simulink model "WMMSupportingForcesGP2020a"  (R2020a)
settings: Solver=ode23t  StartTime=0.0  StopTime=inf  FixedStep=.001  RelTol=1e-3  AbsTol=1e-3
InitFcn:
  | InitializeSimulationGP
  | SimulationParametersGP
values from neighbouring files (symbols this model uses):
  B11_r_B11C = [0.23805608; 0.13201777; 0]    [InitializeSimulationGP.m]
  B11_r_B11Tc1 = [L11; 0; 0]    [InitializeSimulationGP.m]
  B11_Rot_Tc1 = eye(3)    [InitializeSimulationGP.m]
  B11cI = [0.28426000 -0.06487287 0;         -0.06487287  0.54237481 0;                   0  0          0.67891020]    [InitializeSimulationGP.m]
  B12_r_B12C = [0.60504569; 0.27199376; 0.00002484]    [InitializeSimulationGP.m]
  B12_r_B12Tc2 = [L12;0;0]    [InitializeSimulationGP.m]
  B12_Rot_Tc2 = eye(3)    [InitializeSimulationGP.m]
  B12cI = [1.18803886 -2.36786418 0.00280315;          -2.36786418 6.31493281 0.00022322;           0.00280315 0.00022322 7.40915161]    [InitializeSimulationGP.m]
  B31_r_B31C = [0.35781210 0 0]    [InitializeSimulationGP.m]
  B31_Rot_B41 = eye(3)    [InitializeSimulationGP.m]
  B31cI = diag([0.03150902 0.90735702 0.90763033])    [InitializeSimulationGP.m]
  B32_r_B32C = [0.35781210 0 0]    [InitializeSimulationGP.m]
  B32_Rot_B42 = eye(3)    [InitializeSimulationGP.m]
  B32cI = diag([0.03150902 0.90735702 0.90763033])    [InitializeSimulationGP.m]
  B41_r_B41C = [0.55785997 0 0]    [InitializeSimulationGP.m]
  B41_r_B41Tc1 = [lc1;0;0]    [InitializeSimulationGP.m]
  B41cI = diag([0.00370720 0.55759812 0.55785997])    [InitializeSimulationGP.m]
  B42_r_B42C = [0.55785997 0 0]    [InitializeSimulationGP.m]
  B42_r_B42Tc2 = [lc2; 0; 0]    [InitializeSimulationGP.m]
  B42cI = diag([0.00370720 0.55759812 0.55785997])    [InitializeSimulationGP.m]
  B52_r_B52C = [0 0 0.56802906]    [InitializeSimulationGP.m]
  B52_r_B52P32 = [lc3; 0; 0]    [InitializeSimulationGP.m]
  B52_Rot_P32 = eye(3)    [InitializeSimulationGP.m]
  B52cI = diag([0.91789884, 0.91790043, 0.00091463])    [InitializeSimulationGP.m]
  Bc1_r_Bc1B11 = [L1; 0; 0]    [InitializeSimulationGP.m]
  Bc1_r_Bc1B31 = [0;0;0]    [InitializeSimulationGP.m]
  Bc1_r_Bc1C = [0.14178771; 0.16555780; 0]    [InitializeSimulationGP.m]
  Bc1_V = [0;0;0;0;0;0]    [InitializeSimulationGP.m]
  Bc1cI = [+5.892211080 +5.476111360 -0.000019630;          +5.476111360 +28.66965601 -0.000024550;          -0.000019630 -0.000024550 +29.78955950]    [InitializeSimulationGP.m]
  Bc2_r_Bc2B12 = [L2;0;0]    [InitializeSimulationGP.m]
  Bc2_r_Bc2B32 = [0;0;0]    [InitializeSimulationGP.m]
  Bc2_r_Bc2C = [0.54319901; 0.10543875; 0]    [InitializeSimulationGP.m]
  Bc2cI = [0.48071390 0.52924041 0;          0.52924041 5.80912352 0;              0      0          5.97255351]    [InitializeSimulationGP.m]
  BC_r_BCBM = [xCA; yCA; zCA]    [SimulationParametersGP.m]
  BC_Rot_BM = eye(3)    [SimulationParametersGP.m]
  BCI = diag([100 1200 1000])    [SimulationParametersGP.m]
  beta1 = atan2d(374.261,935)*pi/180    [InitializeSimulationGP.m]
  beta2 = atan2d(45.757,373.313)*pi/180    [InitializeSimulationGP.m]
  beta3 = atan2d(139.50,1132.19)*pi/180    [InitializeSimulationGP.m]
  beta4 = atan2d(88.061,296.198)*pi/180    [InitializeSimulationGP.m]
  betaGround = 1e6    (= 1000000)    [SimulationParametersGP.m]
  BFL = 0.05    [SimulationParametersGP.m]
  BFR = 0.05    [SimulationParametersGP.m]
  BM_r_BMBMp = [0;0;0]    [SimulationParametersGP.m]
  BM_Rot_BMp = [cos(gamma) -sin(gamma) 0; sin(gamma) cos(gamma) 0; 0 0 1]    [SimulationParametersGP.m]
  BMp_r_BMpBc1 = [0.185;0;0.205]    [InitializeSimulationGP.m]
  BMp_Rot_Bc1 = [cos(alpha1) -sin(alpha1)  0;                  0            0       -1;                sin(alpha1)  cos(alpha1)  0]    [InitializeSimulationGP.m]
  BRL = 0.05    [SimulationParametersGP.m]
  BRR = 0.05    [SimulationParametersGP.m]
  cc = 0.0    (= 0)    [SimulationParametersGP.m]
  D22F = [0;0;0;0;0;0]    [InitializeSimulationGP.m]
  dT = 0.01    [SimulationParametersGP.m]
  g0 = 9.8066    [SimulationParametersGP.m]
  ground_stiffness = 1e8    (= 100000000)    [SimulationParametersGP.m]
  l1 = 1.15-cc    (= 1.15)    [SimulationParametersGP.m]
  L1 = 1.0071227324212    (= 1.00712273242)    [InitializeSimulationGP.m]
  L11 = 0.37610632101293    (= 0.376106321013)    [InitializeSimulationGP.m]
  L12 = 0.30901132665325    (= 0.309011326653)    [InitializeSimulationGP.m]
  l2 = 1.15+cc    (= 1.15)    [SimulationParametersGP.m]
  L2 = 1.132185817991    (= 1.13218581799)    [InitializeSimulationGP.m]
  lc1 = 0.745    [InitializeSimulationGP.m]
  lc2 = 0.745    [InitializeSimulationGP.m]
  mB11 = 25.52660174    [InitializeSimulationGP.m]
  mB12 = 33.92850233    [InitializeSimulationGP.m]
  mB31 = 17.36281648    [InitializeSimulationGP.m]
  mB32 = 17.36281648    [InitializeSimulationGP.m]
  mB41 = 10.34519231    [InitializeSimulationGP.m]
  mB42 = 10.34519231    [InitializeSimulationGP.m]
  mB52 = 6.73059863    [InitializeSimulationGP.m]
  mBC = 2200    [SimulationParametersGP.m]
  mBc1 = 307.29601379    [InitializeSimulationGP.m]
  mBc2 = 54.58702836    [InitializeSimulationGP.m]
  mFL = 60    [SimulationParametersGP.m]
  mFR = 60    [SimulationParametersGP.m]
  mP22 = 9.26136143    [InitializeSimulationGP.m]
  mP32 = 570.18877059    [InitializeSimulationGP.m]
  mRR = 60    [SimulationParametersGP.m]
  mw = mFL    (= 60)    [SimulationParametersGP.m]
  P22_r_P22C = [0.62192523 0 0]    [InitializeSimulationGP.m]
  P22_Rot_B52 = eye(3)    [InitializeSimulationGP.m]
  P22cI = diag([0.00662754, 1.48387017, 1.48398069])    [InitializeSimulationGP.m]
  P32_r_P32C = [0.25466704; -0.13034397; -0.01302248]    [InitializeSimulationGP.m]
  P32_r_P32D22 = [0.40499744871392; -0.13130517281345; -0.013385243295654]    [InitializeSimulationGP.m]
  P32_Rot_D22 = [1 0 0;              0 0.9707729441837 0.23999977258512;              0 -0.23999977258512 0.9707729441837]    [InitializeSimulationGP.m]
  P32cI = [46.81220713 0.38607676 -0.00453819;          0.38607676 71.92201786 -1.14320993;          -0.00453819 -1.14320993 67.38128576]    [InitializeSimulationGP.m]
  R0FL = 0.35    [SimulationParametersGP.m]
  R0FR = 0.35    [SimulationParametersGP.m]
  R0RL = 0.35    [SimulationParametersGP.m]
  R0RR = 0.35    [SimulationParametersGP.m]
  Rw = R0FL    (= 0.35)    [SimulationParametersGP.m]
  Tc1_r_Tc1Bc2 = [0.098495302558553; 0.01838181329939; 0]    [InitializeSimulationGP.m]
  Tc1_Rot_Bc2 = [cos(alpha2) -sin(alpha2) 0;                sin(alpha2)  cos(alpha2) 0;                0            0           1]    [InitializeSimulationGP.m]
  Tc2_r_Tc2P22 = [-0.048858374920227;0.36587359346146;0.035276938723102]    [InitializeSimulationGP.m]
  Tc2_Rot_P22 = [0.95853460763586 -0.27664713597974  0.0683942111482;                0.28497614981675  0.93051946315663 -0.23004808784757;                0                 0.23999977258511  0.9707729441837]    [InitializeSimulationGP.m]
  Th1A = 10*pi/180    (= 0.174532925199)    [InitializeSimulationGP.m]
  Th1B = 20*pi/180    (= 0.349065850399)    [InitializeSimulationGP.m]
  Th1f = 1    [InitializeSimulationGP.m]
  Th2A = 15*pi/180    (= 0.261799387799)    [InitializeSimulationGP.m]
  Th2B = -70*pi/180    (= -1.2217304764)    [InitializeSimulationGP.m]
  Th2f = 2    [InitializeSimulationGP.m]
  w = wFL    (= 0.875)    [SimulationParametersGP.m]
  W_r_WBc1 = [0.185;0;0.205]    [InitializeSimulationGP.m]
  W_Rot_Bc1 = [cos(alpha1) -sin(alpha1)  0;                  0            0       -1;                sin(alpha1)  cos(alpha1)  0]    [InitializeSimulationGP.m]
  x10 = 0.83    [InitializeSimulationGP.m]
  x20 = 0.83    [InitializeSimulationGP.m]
  x3A = 0.2    [InitializeSimulationGP.m]
  x3B = 0.3    [InitializeSimulationGP.m]
  x3f = 1    [InitializeSimulationGP.m]
  xCA = 0.5    [SimulationParametersGP.m]
  xf = [1;0;0;0;0;0]    [InitializeSimulationGP.m]
  yCA = 0    [SimulationParametersGP.m]
  zC = 0.45    [SimulationParametersGP.m]
  zCA = .25    (= 0.25)    [SimulationParametersGP.m]
  ztau = [0;0;0;0;0;1]    [InitializeSimulationGP.m]
undefined symbols (not defined in the file or in its folder): alphaFL_meas, alphaFR_meas, alphaRL_meas, alphaRR_meas, B11_V, B11Ftot, B12_U_Tc2, B12_V, B12Ftot, B31_r_B31B41, B31_V, B31FTot, B32_r_B32B42, B32_U_B42, B32_V, B32FTot, B41_V, B41FTot, B42_Rot_Tc2, B42_U_Tc2, B42_V, B42FTot, B52_U_P32, B52_V, B52Ftot, Bc1Tot, Bc2_Rot_B12, Bc2_Rot_B32, Bc2_U_B12, Bc2_U_B32, Bc2_V, Bc2Tot, betaC_meas, D22_V, deltaFL_cmd, deltaFL_meas, deltaFR_cmd, deltaFR_meas, deltaRL_cmd, deltaRL_meas, deltaRR_cmd, deltaRR_meas, dOmegaFL_meas, dOmegaFR_meas, dOmegaRL_meas, dOmegaRR_meas, dPsi_meas, dq1, dq11, dq12, dq2, dq21, dq22, dx1, dx2, Floor, FTot_S1, FTot_S2P, FTot_S2R, FzFL ... (+63)
libraries: sm_lib x94, nesl_utility x63, simulink x5
(part 8 of 11)

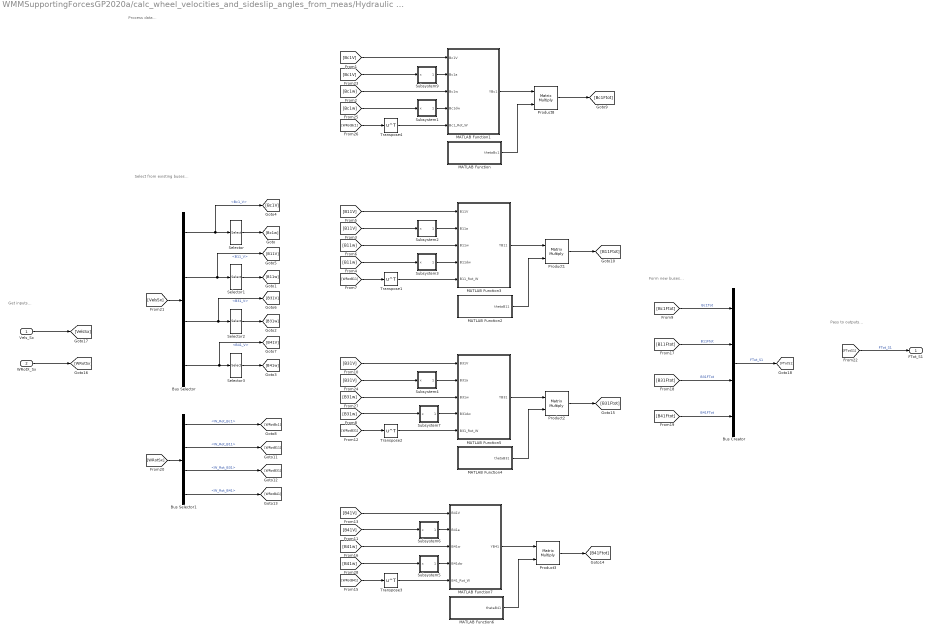
== system WMMSupportingForcesGP2020a/calc_wheel_velocities_and_sideslip_angles_from_meas/Hydraulic manipulator, calculation/AnalyticTotalForces/Structure 1 ==
  note: Pass to outputs...
  note: Get inputs...
  note: Process data...
  note: Form new buses...
  note: Select from existing buses...
  Vels_Sx : Inport
  WRotX_Sx : Inport  Port=2
  Bus Creator : BusCreator  Inputs=Bc1Tot,B11Ftot,B31FTot,B41FTot
  Bus Selector : BusSelector  OutputSignals=Vels_S1.Bc1_V,Vels_S1.B11_V,Vels_S1.B31_V,Vels_S1.B41_V
  Bus Selector1 : BusSelector  OutputSignals=WRotX_S1.W_Rot_Bc1,WRotX_S1.W_Rot_B11,WRotX_S1.W_Rot_B31,WRotX_S1.W_Rot_B41
  MATLAB Function : MATLAB Function  TreatAsAtomicUnit=on
  MATLAB Function1 : MATLAB Function  TreatAsAtomicUnit=on
  MATLAB Function2 : MATLAB Function  TreatAsAtomicUnit=on
  MATLAB Function3 : MATLAB Function  TreatAsAtomicUnit=on
  MATLAB Function4 : MATLAB Function  TreatAsAtomicUnit=on
  MATLAB Function5 : MATLAB Function  TreatAsAtomicUnit=on
  MATLAB Function6 : MATLAB Function  TreatAsAtomicUnit=on
  MATLAB Function7 : MATLAB Function  TreatAsAtomicUnit=on
  Product{1..3,8} (4 alike) : Product  Multiplication=Matrix(*)
  Selector{,1..3} (4 alike) : Selector  InputPortWidth=6  IndexOptions=Index vector (dialog)  Indices=[4 5 6]  OutputSizes=1
  Subsystem1 : Subsystem
  Subsystem2 : Subsystem
  Subsystem3 : Subsystem
  Subsystem4 : Subsystem
  Subsystem5 : Subsystem
  Subsystem6 : Subsystem
  Subsystem7 : Subsystem
  Subsystem9 : Subsystem
  Transpose{1..4} (4 alike) : Math  Operator=transpose  SaturateOnIntegerOverflow=on
  FTot_S1 : Outport
  wires:
  Bus Selector/4 -> Selector3/1, [B41V]  "<B41_V>"
  Bus Selector1/3 -> [WRotB31]  "<W_Rot_B31>"
  Bus Selector1/1 -> [WRotBc1]  "<W_Rot_Bc1>"
  [B11Ftot] -> Bus Creator/2  "B11Ftot"
  [WRotB31] -> Transpose2/1
  Selector/1 -> [Bc1w]
  Selector3/1 -> [B41w]
  Bus Selector/3 -> Selector2/1, [B31V]  "<B31_V>"
  [B31Ftot] -> Bus Creator/3  "B31FTot"
  Bus Selector/1 -> Selector/1, [Bc1V]  "<Bc1_V>"
  Bus Selector/2 -> Selector1/1, [B11V]  "<B11_V>"
  [B41Ftot] -> Bus Creator/4  "B41FTot"
  Selector2/1 -> [B31w]
  [Bc1Ftot] -> Bus Creator/1  "Bc1Tot"
  Bus Selector1/2 -> [WRotB11]  "<W_Rot_B11>"
  [WRotB11] -> Transpose1/1
  Bus Selector1/4 -> [WRotB41]  "<W_Rot_B41>"
  WRotX_Sx/1 -> [WRotSx]
  [WRotSx] -> Bus Selector1/1
  Vels_Sx/1 -> [VelsSx]
  [VelsSx] -> Bus Selector/1
  Bus Creator/1 -> [FTotS1]  "FTot_S1"
  [FTotS1] -> FTot_S1/1  "FTot_S1"
  Selector1/1 -> [B11w]
  [WRotBc1] -> Transpose4/1
  Transpose4/1 -> MATLAB Function1/5(Bc1_Rot_W)
  Subsystem1/1(dx/dt) -> MATLAB Function1/4(Bc1dw)
  [Bc1w] -> Subsystem1/1(x)
  [Bc1V] -> Subsystem9/1(x)
  Subsystem9/1(dx/dt) -> MATLAB Function1/2(Bc1a)
  MATLAB Function1/1(YBc1) -> Product8/1
  MATLAB Function/1(thetaBc1) -> Product8/2
  Product8/1 -> [Bc1Ftot]
  [Bc1V] -> MATLAB Function1/1(Bc1V)
  [Bc1w] -> MATLAB Function1/3(Bc1w)
  [B11w] -> MATLAB Function3/3(B11w)
  [B11V] -> MATLAB Function3/1(B11V)
  MATLAB Function2/1(thetaB11) -> Product1/2
  MATLAB Function3/1(YB11) -> Product1/1
  Subsystem2/1(dx/dt) -> MATLAB Function3/2(B11a)
  [B11V] -> Subsystem2/1(x)
  [B11w] -> Subsystem3/1(x)
  Subsystem3/1(dx/dt) -> MATLAB Function3/4(B11dw)
  Transpose1/1 -> MATLAB Function3/5(B11_Rot_W)
  Product1/1 -> [B11Ftot]
  Product2/1 -> [B31Ftot]
  Transpose2/1 -> MATLAB Function5/5(B31_Rot_W)
  Subsystem7/1(dx/dt) -> MATLAB Function5/4(B31dw)
  [B31w] -> Subsystem7/1(x)
  [B31V] -> Subsystem4/1(x)
  Subsystem4/1(dx/dt) -> MATLAB Function5/2(B31a)
  MATLAB Function5/1(YB31) -> Product2/1
  MATLAB Function4/1(thetaB31) -> Product2/2
  [B31V] -> MATLAB Function5/1(B31V)
  [B31w] -> MATLAB Function5/3(B31w)
  [B41w] -> MATLAB Function7/3(B41w)
  [B41V] -> MATLAB Function7/1(B41V)
  MATLAB Function6/1(thetaB41) -> Product3/2
  MATLAB Function7/1(YB41) -> Product3/1
  Subsystem6/1(dx/dt) -> MATLAB Function7/2(B41a)
  [B41V] -> Subsystem6/1(x)
  [B41w] -> Subsystem5/1(x)
  Subsystem5/1(dx/dt) -> MATLAB Function7/4(B41dw)
  Transpose3/1 -> MATLAB Function7/5(B41_Rot_W)
  Product3/1 -> [B41Ftot]
  [WRotB41] -> Transpose3/1

== system WMMSupportingForcesGP2020a/calc_wheel_velocities_and_sideslip_angles_from_meas/Hydraulic manipulator, calculation/AnalyticTotalForces/Structure 2 (Prismatic segment) ==
  note: Select from existing buses...
  note: Form new buses...
  note: Get inputs...
  note: Pass to outputs...
  note: Process data...
  Vels_Sx : Inport
  WRotX_Sx : Inport  Port=2
  Bus Creator : BusCreator  Inputs=P22FTot,B52Ftot,P32FTot
  Bus Selector : BusSelector  OutputSignals=Vels_S2R.P22_V,Vels_S2P.B52_V,Vels_S2P.P32_V
  Bus Selector1 : BusSelector  OutputSignals=WRotX_S2R.W_Rot_P22,WRotX_S2P.W_Rot_B52,WRotX_S2P.W_Rot_P32
  MATLAB Function1 : MATLAB Function  TreatAsAtomicUnit=on
  MATLAB Function2 : MATLAB Function  TreatAsAtomicUnit=on
  MATLAB Function3 : MATLAB Function  TreatAsAtomicUnit=on
  MATLAB Function4 : MATLAB Function  TreatAsAtomicUnit=on
  MATLAB Function6 : MATLAB Function  TreatAsAtomicUnit=on
  MATLAB Function7 : MATLAB Function  TreatAsAtomicUnit=on
  Product1 : Product  Multiplication=Matrix(*)
  Product2 : Product  Multiplication=Matrix(*)
  Product3 : Product  Multiplication=Matrix(*)
  Selector : Selector  InputPortWidth=6  IndexOptions=Index vector (dialog)  Indices=[4 5 6]  OutputSizes=1
  Selector1 : Selector  InputPortWidth=6  IndexOptions=Index vector (dialog)  Indices=[4 5 6]  OutputSizes=1
  Selector2 : Selector  InputPortWidth=6  IndexOptions=Index vector (dialog)  Indices=[4 5 6]  OutputSizes=1
  Subsystem1 : Subsystem
  Subsystem2 : Subsystem
  Subsystem3 : Subsystem
  Subsystem4 : Subsystem
  Subsystem5 : Subsystem
  Subsystem6 : Subsystem
  Transpose : Math  Operator=transpose  SaturateOnIntegerOverflow=on
  Transpose1 : Math  Operator=transpose  SaturateOnIntegerOverflow=on
  Transpose2 : Math  Operator=transpose  SaturateOnIntegerOverflow=on
  FTot_S2P : Outport
  wires:
  [FTotS2P] -> FTot_S2P/1  "FTot_S2P"
  WRotX_Sx/1 -> [WRotSx]
  Vels_Sx/1 -> [VelsSx]
  Product3/1 -> [P32Ftot]
  Bus Selector1/3 -> [WRotP32]  "<W_Rot_P32>"
  [VelsSx] -> Bus Selector/1
  Product2/1 -> [B52Ftot]
  Bus Selector1/1 -> [WRotP22]  "<W_Rot_P22>"
  [B52Ftot] -> Bus Creator/2  "B52Ftot"
  Product1/1 -> [P22Ftot]
  [WRotP22] -> Transpose/1
  [WRotP32] -> Transpose2/1
  Selector/1 -> [P22w]
  Bus Creator/1 -> [FTotS2P]
  [WRotSx] -> Bus Selector1/1
  Selector1/1 -> [B52w]
  [P32Ftot] -> Bus Creator/3  "P32FTot"
  Selector2/1 -> [P32w]
  [P22Ftot] -> Bus Creator/1  "P22FTot"
  Bus Selector1/2 -> [WRotB52]  "<W_Rot_B52>"
  Bus Selector/1 -> [P22V], Selector/1  "<P22_V>"
  Bus Selector/3 -> [P32V], Selector2/1  "<P32_V>"
  Bus Selector/2 -> [B52V], Selector1/1  "<B52_V>"
  [P22V] -> MATLAB Function7/1(P22V)
  Transpose/1 -> MATLAB Function7/5(P22_Rot_W)
  [P22V] -> Subsystem2/1(x)
  [P22w] -> Subsystem1/1(x)
  MATLAB Function7/1(YP22) -> Product1/1
  Subsystem1/1(dx/dt) -> MATLAB Function7/4(P22dw)
  MATLAB Function6/1(thetaP22) -> Product1/2
  Subsystem2/1(dx/dt) -> MATLAB Function7/2(P22a)
  [P22w] -> MATLAB Function7/3(P22w)
  MATLAB Function1/1(thetaB52) -> Product2/2
  MATLAB Function2/1(YB52) -> Product2/1
  [WRotB52] -> Transpose1/1
  [B52V] -> MATLAB Function2/1(B52V)
  [B52V] -> Subsystem3/1(x)
  Subsystem3/1(dx/dt) -> MATLAB Function2/2(B52a)
  [B52w] -> MATLAB Function2/3(B52w)
  [B52w] -> Subsystem4/1(x)
  Subsystem4/1(dx/dt) -> MATLAB Function2/4(B52dw)
  Transpose1/1 -> MATLAB Function2/5(B52_Rot_W)
  Transpose2/1 -> MATLAB Function4/5(P32_Rot_W)
  Subsystem6/1(dx/dt) -> MATLAB Function4/4(P32dw)
  [P32w] -> Subsystem6/1(x)
  [P32w] -> MATLAB Function4/3(P32w)
  Subsystem5/1(dx/dt) -> MATLAB Function4/2(P32a)
  [P32V] -> Subsystem5/1(x)
  [P32V] -> MATLAB Function4/1(P32V)
  MATLAB Function4/1(YP32) -> Product3/1
  MATLAB Function3/1(thetaP32) -> Product3/2

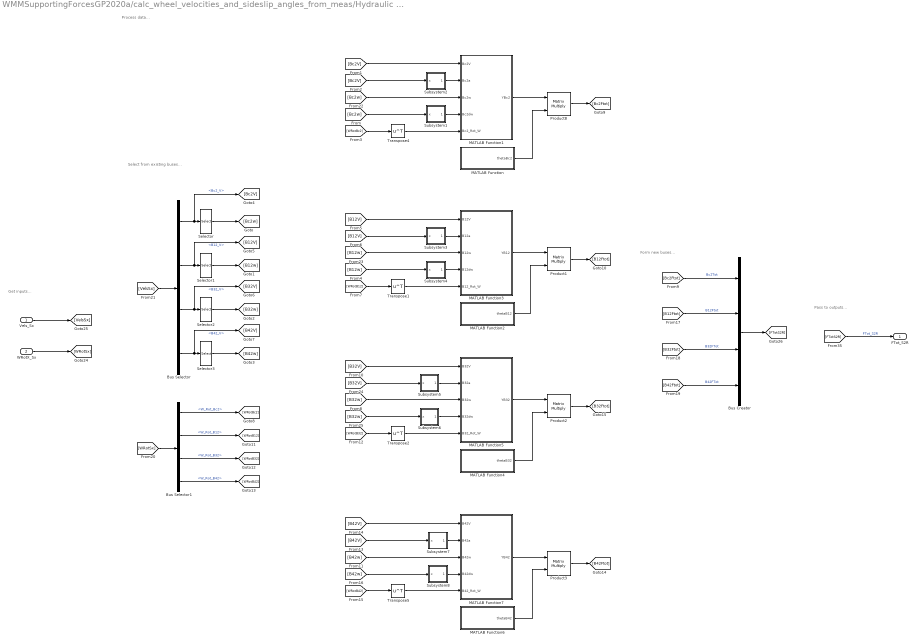
== system WMMSupportingForcesGP2020a/calc_wheel_velocities_and_sideslip_angles_from_meas/Hydraulic manipulator, calculation/AnalyticTotalForces/Structure 2 (Revolute segment) ==
  note: Process data...
  note: Pass to outputs...
  note: Get inputs...
  note: Form new buses...
  note: Select from existing buses...
  Vels_Sx : Inport
  WRotX_Sx : Inport  Port=2
  Bus Creator : BusCreator  Inputs=Bc2Tot,B12Ftot,B32FTot,B42FTot
  Bus Selector : BusSelector  OutputSignals=Vels_S1.Bc2_V,Vels_S2R.B12_V,Vels_S2R.B32_V,Vels_S2R.B42_V
  Bus Selector1 : BusSelector  OutputSignals=WRotX_S1.W_Rot_Bc2,WRotX_S2R.W_Rot_B12,WRotX_S2R.W_Rot_B32,WRotX_S2R.W_Rot_B42
  MATLAB Function : MATLAB Function  TreatAsAtomicUnit=on
  MATLAB Function1 : MATLAB Function  TreatAsAtomicUnit=on
  MATLAB Function2 : MATLAB Function  TreatAsAtomicUnit=on
  MATLAB Function3 : MATLAB Function  TreatAsAtomicUnit=on
  MATLAB Function4 : MATLAB Function  TreatAsAtomicUnit=on
  MATLAB Function5 : MATLAB Function  TreatAsAtomicUnit=on
  MATLAB Function6 : MATLAB Function  TreatAsAtomicUnit=on
  MATLAB Function7 : MATLAB Function  TreatAsAtomicUnit=on
  Product{1..3,8} (4 alike) : Product  Multiplication=Matrix(*)
  Selector{,1..3} (4 alike) : Selector  InputPortWidth=6  IndexOptions=Index vector (dialog)  Indices=[4 5 6]  OutputSizes=1
  Subsystem1 : Subsystem
  Subsystem2 : Subsystem
  Subsystem3 : Subsystem
  Subsystem4 : Subsystem
  Subsystem5 : Subsystem
  Subsystem6 : Subsystem
  Subsystem7 : Subsystem
  Subsystem8 : Subsystem
  Transpose{1..2,4..5} (4 alike) : Math  Operator=transpose  SaturateOnIntegerOverflow=on
  FTot_S2R : Outport
  wires:
  Bus Selector1/4 -> [WRotB42]  "<W_Rot_B42>"
  [WRotB12] -> Transpose1/1
  Bus Selector1/2 -> [WRotB12]  "<W_Rot_B12>"
  [WRotB42] -> Transpose5/1
  [Bc2Ftot] -> Bus Creator/1  "Bc2Tot"
  Selector2/1 -> [B32w]
  [B42Ftot] -> Bus Creator/4  "B42FTot"
  Bus Selector/2 -> Selector1/1, [B12V]  "<B12_V>"
  Bus Selector/1 -> Selector/1, [Bc2V]  "<Bc2_V>"
  [B32Ftot] -> Bus Creator/3  "B32FTot"
  Bus Selector/3 -> Selector2/1, [B32V]  "<B32_V>"
  Selector1/1 -> [B12w]
  [WRotSx] -> Bus Selector1/1
  Selector3/1 -> [B42w]
  Bus Creator/1 -> [FTotS2R]
  Selector/1 -> [Bc2w]
  [WRotB32] -> Transpose2/1
  Product3/1 -> [B42Ftot]
  Product8/1 -> [Bc2Ftot]
  [B12Ftot] -> Bus Creator/2  "B12Ftot"
  Bus Selector1/1 -> [WRotBc2]  "<W_Rot_Bc2>"
  [VelsSx] -> Bus Selector/1
  Bus Selector1/3 -> [WRotB32]  "<W_Rot_B32>"
  Bus Selector/4 -> Selector3/1, [B42V]  "<B42_V>"
  Vels_Sx/1 -> [VelsSx]
  WRotX_Sx/1 -> [WRotSx]
  [FTotS2R] -> FTot_S2R/1  "FTot_S2R"
  [Bc2w] -> Subsystem1/1(x)
  [Bc2w] -> MATLAB Function1/3(Bc2w)
  [WRotBc2] -> Transpose4/1
  Transpose4/1 -> MATLAB Function1/5(Bc2_Rot_W)
  Subsystem1/1(dx/dt) -> MATLAB Function1/4(Bc2dw)
  [Bc2V] -> MATLAB Function1/1(Bc2V)
  MATLAB Function/1(thetaBc2) -> Product8/2
  [Bc2V] -> Subsystem2/1(x)
  MATLAB Function1/1(YBc2) -> Product8/1
  Subsystem2/1(dx/dt) -> MATLAB Function1/2(Bc2a)
  Subsystem3/1(dx/dt) -> MATLAB Function3/2(B12a)
  MATLAB Function3/1(YB12) -> Product1/1
  [B12V] -> Subsystem3/1(x)
  MATLAB Function2/1(thetaB12) -> Product1/2
  [B12V] -> MATLAB Function3/1(B12V)
  Subsystem4/1(dx/dt) -> MATLAB Function3/4(B12dw)
  Transpose1/1 -> MATLAB Function3/5(B12_Rot_W)
  [B12w] -> MATLAB Function3/3(B12w)
  [B12w] -> Subsystem4/1(x)
  Product1/1 -> [B12Ftot]
  [B32w] -> Subsystem6/1(x)
  [B32w] -> MATLAB Function5/3(B32w)
  Subsystem6/1(dx/dt) -> MATLAB Function5/4(B32dw)
  [B32V] -> MATLAB Function5/1(B32V)
  MATLAB Function4/1(thetaB32) -> Product2/2
  [B32V] -> Subsystem5/1(x)
  MATLAB Function5/1(YB32) -> Product2/1
  Subsystem5/1(dx/dt) -> MATLAB Function5/2(B32a)
  Transpose2/1 -> MATLAB Function5/5(B32_Rot_W)
  Product2/1 -> [B32Ftot]
  Transpose5/1 -> MATLAB Function7/5(B42_Rot_W)
  Subsystem7/1(dx/dt) -> MATLAB Function7/2(B42a)
  MATLAB Function7/1(YB42) -> Product3/1
  [B42V] -> Subsystem7/1(x)
  MATLAB Function6/1(thetaB42) -> Product3/2
  [B42V] -> MATLAB Function7/1(B42V)
  Subsystem8/1(dx/dt) -> MATLAB Function7/4(B42dw)
  [B42w] -> MATLAB Function7/3(B42w)
  [B42w] -> Subsystem8/1(x)

== system WMMSupportingForcesGP2020a/calc_wheel_velocities_and_sideslip_angles_from_meas/Hydraulic manipulator, calculation/AnalyticVelocities/Structure 1 ==
  note: Pass to outputs...
  note: Process data...
  note: Calculate geometric properties of the closed kinematic chain 1...
  note: Get inputs...
  note: Form relevant position vectors...
  note: Form relevant rotation matrices...
  note: Form relevant velocity/force transformation matrices...
  note: Form relevant linear/angular velocities...
  q1[rad] : Inport  Unit=rad
  W_Rot_Bc1 : Inport  Port=2
  Bc1_V : Inport  Port=3  PortDimensions=[6 1]
  GeomPropS1 : Subsystem
  PosVecsS1 : Subsystem
  RotMatsS1 : Subsystem
  UMatsS1 : Subsystem
  VelsS1 : Subsystem
  Geom_S1 : Outport
  PosVecs_S1 : Outport  Port=2
  WRotX_S1 : Outport  Port=3
  Vels_S1 : Outport  Port=4
  UMat_S1 : Outport  Port=5
  wires:
  GeomPropS1/1(GeomProp_S1) -> [GeomS1]
  [GeomS1] -> PosVecsS1/1(GeomProp_CC1)
  [GeomS1] -> RotMatsS1/1(GeomProp_S1)
  [GeomS1] -> VelsS1/1(GeomProp_S1)
  RotMatsS1/1(RotMats_S1) -> [RotMatsS1]
  [RotMatsS1] -> UMatsS1/2(RotMats_S1)
  PosVecsS1/1(PosVecs_S1) -> [PosVecsS1]
  [PosVecsS1] -> UMatsS1/1(PosVecs_S1)
  [GeomS1] -> Geom_S1/1
  VelsS1/1(Vels_S1) -> [VelsS1]
  [VelsS1] -> Vels_S1/1
  UMatsS1/1(UMat_S1) -> [UMatsS1]
  [UMatsS1] -> VelsS1/2(UMats_S1)
  Bc1_V/1 -> [Bc1V]  "Bc1V"
  [Bc1V] -> VelsS1/3(Bc1_V)
  W_Rot_Bc1/1 -> [WRotBc1]  "WRotBc1"
  [WRotBc1] -> RotMatsS1/2(WRotBc1)
  [UMatsS1] -> UMat_S1/1
  RotMatsS1/2(WRotX_S1) -> [WRotXS1]
  [WRotXS1] -> WRotX_S1/1
  q1[rad]/1 -> [q1]  "q1"
  [q1] -> GeomPropS1/1(q1)
  [PosVecsS1] -> PosVecs_S1/1

== system WMMSupportingForcesGP2020a/calc_wheel_velocities_and_sideslip_angles_from_meas/Hydraulic manipulator, calculation/AnalyticVelocities/Structure 2 (Prismatic segment) ==
  note: Pass to outputs...
  note: Get inputs...
  note: Process data...
  x3 : Inport
  WRotX_S2R : Inport  Port=2
  Vels_S2R : Inport  Port=3
  GeomPropS2P : Subsystem
  PosVecsS2P : Subsystem
  RotMatsS2P : Subsystem
  UMatsS2P : Subsystem
  VelsS2P : Subsystem
  GeomProp_S2P : Outport
  PosVecs_S2P : Outport  Port=2
  WRotX_S2P : Outport  Port=3
  Vels_S2P : Outport  Port=4
  UMats_S2P : Outport  Port=5
  wires:
  x3/1 -> [x3]
  Vels_S2R/1 -> [VelsS2R]
  WRotX_S2R/1 -> [WRotXS2R]
  GeomPropS2P/1(GeomProp_S2P) -> [GeomS2P]
  [GeomS2P] -> GeomProp_S2P/1
  [x3] -> GeomPropS2P/1(x3)
  PosVecsS2P/1(PosVecsS2P) -> [PosVecsS2P]
  [x3] -> PosVecsS2P/1(x3)
  [PosVecsS2P] -> PosVecs_S2P/1
  RotMatsS2P/2(WRotX_S2P) -> [WRotXS2P]
  [WRotXS2R] -> RotMatsS2P/1(WRotX_S2R)
  [WRotXS2P] -> WRotX_S2P/1
  RotMatsS2P/1(RotMats_S2P) -> [RotMatsS2P]
  [PosVecsS2P] -> UMatsS2P/1(PosVecs_S2P)
  [RotMatsS2P] -> UMatsS2P/2(RotMats_S2P)
  UMatsS2P/1(UMats_S2P) -> [UMatsS2P]
  [UMatsS2P] -> UMats_S2P/1
  [VelsS2R] -> VelsS2P/3(Vels_S2R)
  [GeomS2P] -> VelsS2P/1(GeomProp_S2P)
  [UMatsS2P] -> VelsS2P/2(UMats_S2P)
  VelsS2P/1(Vels_S2P) -> [VelsS2P]
  [VelsS2P] -> Vels_S2P/1

== system WMMSupportingForcesGP2020a/calc_wheel_velocities_and_sideslip_angles_from_meas/Hydraulic manipulator, calculation/AnalyticVelocities/Structure 2 (Revolute segment) ==
  note: Pass to outputs...
  note: Process data...
  note: Get inputs...
  q2[rad] : Inport
  WRotX_S1 : Inport  Port=2
  Vels_S1 : Inport  Port=3
  GeomPropS2R : Subsystem
  PosVecsS2R : Subsystem
  RotMatsS2R : Subsystem
  UMatS2R : Subsystem
  VelsS2R : Subsystem
  GeomProp_S2R : Outport
  PosVecs_S2R : Outport  Port=2
  WRotX_S2R : Outport  Port=3
  Vels_S2R : Outport  Port=4
  UMats_S2R : Outport  Port=5
  wires:
  [GeomS2R] -> VelsS2R/1(GeomProp_CC2)
  [GeomS2R] -> RotMatsS2R/1(GeomProp_CC2)
  [GeomS2R] -> PosVecsS2R/1(GeomProp_S2R)
  GeomPropS2R/1(GeomProp_S2R) -> [GeomS2R]
  [q2] -> GeomPropS2R/1(q2)
  [GeomS2R] -> GeomProp_S2R/1  "GeomS2R"
  RotMatsS2R/1(RotMats_S2) -> [RotMatsS2R]
  q2[rad]/1 -> [q2]  "q2"
  PosVecsS2R/1(PosVecs_S2) -> [PosVecsS2R]
  [PosVecsS2R] -> UMatS2R/1(PosVecs_S2)
  [PosVecsS2R] -> PosVecs_S2R/1  "PosVecsS2R"
  [RotMatsS2R] -> UMatS2R/2(RotMats_S2)
  UMatS2R/1(UMatS2) -> [UMatsS2R]
  [UMatsS2R] -> VelsS2R/2(UMats_S2)
  [UMatsS2R] -> UMats_S2R/1  "UMatsS2R"
  RotMatsS2R/2(WRotX_S2) -> [WRotXS2R]
  [WRotXS2R] -> WRotX_S2R/1  "WRotXS2R"
  Vels_S1/1 -> [VelsS1]  "Vels_S1"
  [VelsS1] -> VelsS2R/3(Vels_S1)
  WRotX_S1/1 -> [WRotXS1]  "WRotX_S1"
  [WRotXS1] -> RotMatsS2R/2(WRotX_S1)
  VelsS2R/1(Vels_S2) -> [VelsS2R]
  [VelsS2R] -> Vels_S2R/1  "VelsS2R"

== system WMMSupportingForcesGP2020a/calc_wheel_velocities_and_sideslip_angles_from_meas/Hydraulic manipulator, calculation/AnalyticTotalForces/Structure 1/Subsystem1 ==
  x : Inport
  Demux : Demux  Outputs=3
  Mux : Mux  Inputs=3
  Subsystem1 : Subsystem
  Subsystem2 : Subsystem
  Subsystem3 : Subsystem
  dx/dt : Outport
  wires:
  x/1 -> Demux/1
  Demux/3 -> Subsystem3/1(x)
  Demux/2 -> Subsystem2/1(x)
  Demux/1 -> Subsystem1/1(x)
  Subsystem3/1(dx/dt) -> Mux/3
  Subsystem2/1(dx/dt) -> Mux/2
  Subsystem1/1(dx/dt) -> Mux/1
  Mux/1 -> dx/dt/1

== system WMMSupportingForcesGP2020a/calc_wheel_velocities_and_sideslip_angles_from_meas/Hydraulic manipulator, calculation/AnalyticTotalForces/Structure 1/Subsystem2 ==
  x : Inport
  Demux : Demux  Outputs=6
  Mux : Mux  Inputs=6
  Subsystem1 : Subsystem
  Subsystem2 : Subsystem
  Subsystem3 : Subsystem
  Subsystem4 : Subsystem
  Subsystem5 : Subsystem
  Subsystem6 : Subsystem
  dx/dt : Outport
  wires:
  x/1 -> Demux/1
  Demux/6 -> Subsystem6/1(x)
  Demux/5 -> Subsystem5/1(x)
  Demux/4 -> Subsystem4/1(x)
  Demux/3 -> Subsystem3/1(x)
  Demux/2 -> Subsystem2/1(x)
  Demux/1 -> Subsystem1/1(x)
  Subsystem6/1(dx/dt) -> Mux/6
  Subsystem5/1(dx/dt) -> Mux/5
  Subsystem4/1(dx/dt) -> Mux/4
  Subsystem3/1(dx/dt) -> Mux/3
  Subsystem2/1(dx/dt) -> Mux/2
  Subsystem1/1(dx/dt) -> Mux/1
  Mux/1 -> dx/dt/1

== system WMMSupportingForcesGP2020a/calc_wheel_velocities_and_sideslip_angles_from_meas/Hydraulic manipulator, calculation/AnalyticTotalForces/Structure 1/Subsystem3 ==
  x : Inport
  Demux : Demux  Outputs=3
  Mux : Mux  Inputs=3
  Subsystem1 : Subsystem
  Subsystem2 : Subsystem
  Subsystem3 : Subsystem
  dx/dt : Outport
  wires:
  x/1 -> Demux/1
  Demux/3 -> Subsystem3/1(x)
  Demux/2 -> Subsystem2/1(x)
  Demux/1 -> Subsystem1/1(x)
  Subsystem3/1(dx/dt) -> Mux/3
  Subsystem2/1(dx/dt) -> Mux/2
  Subsystem1/1(dx/dt) -> Mux/1
  Mux/1 -> dx/dt/1

== system WMMSupportingForcesGP2020a/calc_wheel_velocities_and_sideslip_angles_from_meas/Hydraulic manipulator, calculation/AnalyticTotalForces/Structure 1/Subsystem4 ==
  x : Inport
  Demux : Demux  Outputs=6
  Mux : Mux  Inputs=6
  Subsystem1 : Subsystem
  Subsystem2 : Subsystem
  Subsystem3 : Subsystem
  Subsystem4 : Subsystem
  Subsystem5 : Subsystem
  Subsystem6 : Subsystem
  dx/dt : Outport
  wires:
  x/1 -> Demux/1
  Demux/6 -> Subsystem6/1(x)
  Demux/5 -> Subsystem5/1(x)
  Demux/4 -> Subsystem4/1(x)
  Demux/3 -> Subsystem3/1(x)
  Demux/2 -> Subsystem2/1(x)
  Demux/1 -> Subsystem1/1(x)
  Subsystem6/1(dx/dt) -> Mux/6
  Subsystem5/1(dx/dt) -> Mux/5
  Subsystem4/1(dx/dt) -> Mux/4
  Subsystem3/1(dx/dt) -> Mux/3
  Subsystem2/1(dx/dt) -> Mux/2
  Subsystem1/1(dx/dt) -> Mux/1
  Mux/1 -> dx/dt/1

== system WMMSupportingForcesGP2020a/calc_wheel_velocities_and_sideslip_angles_from_meas/Hydraulic manipulator, calculation/AnalyticTotalForces/Structure 1/Subsystem5 ==
  x : Inport
  Demux : Demux  Outputs=3
  Mux : Mux  Inputs=3
  Subsystem1 : Subsystem
  Subsystem2 : Subsystem
  Subsystem3 : Subsystem
  dx/dt : Outport
  wires:
  x/1 -> Demux/1
  Demux/3 -> Subsystem3/1(x)
  Demux/2 -> Subsystem2/1(x)
  Demux/1 -> Subsystem1/1(x)
  Subsystem3/1(dx/dt) -> Mux/3
  Subsystem2/1(dx/dt) -> Mux/2
  Subsystem1/1(dx/dt) -> Mux/1
  Mux/1 -> dx/dt/1

== system WMMSupportingForcesGP2020a/calc_wheel_velocities_and_sideslip_angles_from_meas/Hydraulic manipulator, calculation/AnalyticTotalForces/Structure 1/Subsystem6 ==
  x : Inport
  Demux : Demux  Outputs=6
  Mux : Mux  Inputs=6
  Subsystem1 : Subsystem
  Subsystem2 : Subsystem
  Subsystem3 : Subsystem
  Subsystem4 : Subsystem
  Subsystem5 : Subsystem
  Subsystem6 : Subsystem
  dx/dt : Outport
  wires:
  x/1 -> Demux/1
  Demux/6 -> Subsystem6/1(x)
  Demux/5 -> Subsystem5/1(x)
  Demux/4 -> Subsystem4/1(x)
  Demux/3 -> Subsystem3/1(x)
  Demux/2 -> Subsystem2/1(x)
  Demux/1 -> Subsystem1/1(x)
  Subsystem6/1(dx/dt) -> Mux/6
  Subsystem5/1(dx/dt) -> Mux/5
  Subsystem4/1(dx/dt) -> Mux/4
  Subsystem3/1(dx/dt) -> Mux/3
  Subsystem2/1(dx/dt) -> Mux/2
  Subsystem1/1(dx/dt) -> Mux/1
  Mux/1 -> dx/dt/1

== system WMMSupportingForcesGP2020a/calc_wheel_velocities_and_sideslip_angles_from_meas/Hydraulic manipulator, calculation/AnalyticTotalForces/Structure 1/Subsystem7 ==
  x : Inport
  Demux : Demux  Outputs=3
  Mux : Mux  Inputs=3
  Subsystem1 : Subsystem
  Subsystem2 : Subsystem
  Subsystem3 : Subsystem
  dx/dt : Outport
  wires:
  x/1 -> Demux/1
  Demux/3 -> Subsystem3/1(x)
  Demux/2 -> Subsystem2/1(x)
  Demux/1 -> Subsystem1/1(x)
  Subsystem3/1(dx/dt) -> Mux/3
  Subsystem2/1(dx/dt) -> Mux/2
  Subsystem1/1(dx/dt) -> Mux/1
  Mux/1 -> dx/dt/1

== system WMMSupportingForcesGP2020a/calc_wheel_velocities_and_sideslip_angles_from_meas/Hydraulic manipulator, calculation/AnalyticTotalForces/Structure 1/Subsystem9 ==
  x : Inport
  Demux : Demux  Outputs=6
  Mux : Mux  Inputs=6
  Subsystem1 : Subsystem
  Subsystem2 : Subsystem
  Subsystem3 : Subsystem
  Subsystem4 : Subsystem
  Subsystem5 : Subsystem
  Subsystem6 : Subsystem
  dx/dt : Outport
  wires:
  x/1 -> Demux/1
  Demux/6 -> Subsystem6/1(x)
  Demux/5 -> Subsystem5/1(x)
  Demux/4 -> Subsystem4/1(x)
  Demux/3 -> Subsystem3/1(x)
  Demux/2 -> Subsystem2/1(x)
  Demux/1 -> Subsystem1/1(x)
  Subsystem6/1(dx/dt) -> Mux/6
  Subsystem5/1(dx/dt) -> Mux/5
  Subsystem4/1(dx/dt) -> Mux/4
  Subsystem3/1(dx/dt) -> Mux/3
  Subsystem2/1(dx/dt) -> Mux/2
  Subsystem1/1(dx/dt) -> Mux/1
  Mux/1 -> dx/dt/1

== system WMMSupportingForcesGP2020a/calc_wheel_velocities_and_sideslip_angles_from_meas/Hydraulic manipulator, calculation/AnalyticTotalForces/Structure 2 (Prismatic segment)/Subsystem1 ==
  x : Inport
  Delay : Delay  DelayLength=1  InitialConditionSource=Input port
      settings: InputPortMap=u0,p4
  Gain8 : Gain  Gain=1/dT
  Rate Transition : RateTransition  OutPortSampleTime=dT
  Rate Transition1 : RateTransition
  Sum4 : Sum  Inputs=|+-
  dx/dt : Outport
  wires:
  Rate Transition/1 -> Delay/2, Delay/1, Sum4/1
  Sum4/1 -> Gain8/1
  Gain8/1 -> Rate Transition1/1
  Delay/1 -> Sum4/2
  x/1 -> Rate Transition/1
  Rate Transition1/1 -> dx/dt/1

== system WMMSupportingForcesGP2020a/calc_wheel_velocities_and_sideslip_angles_from_meas/Hydraulic manipulator, calculation/AnalyticTotalForces/Structure 2 (Prismatic segment)/Subsystem2 ==
  x : Inport
  Delay : Delay  DelayLength=1  InitialConditionSource=Input port
      settings: InputPortMap=u0,p4
  Gain8 : Gain  Gain=1/dT
  Rate Transition : RateTransition  OutPortSampleTime=dT
  Rate Transition1 : RateTransition
  Sum4 : Sum  Inputs=|+-
  dx/dt : Outport
  wires:
  Rate Transition/1 -> Delay/2, Delay/1, Sum4/1
  Sum4/1 -> Gain8/1
  Gain8/1 -> Rate Transition1/1
  Delay/1 -> Sum4/2
  x/1 -> Rate Transition/1
  Rate Transition1/1 -> dx/dt/1

== system WMMSupportingForcesGP2020a/calc_wheel_velocities_and_sideslip_angles_from_meas/Hydraulic manipulator, calculation/AnalyticTotalForces/Structure 2 (Prismatic segment)/Subsystem3 ==
  x : Inport
  Delay : Delay  DelayLength=1  InitialConditionSource=Input port
      settings: InputPortMap=u0,p4
  Gain8 : Gain  Gain=1/dT
  Rate Transition : RateTransition  OutPortSampleTime=dT
  Rate Transition1 : RateTransition
  Sum4 : Sum  Inputs=|+-
  dx/dt : Outport
  wires:
  Rate Transition/1 -> Delay/2, Delay/1, Sum4/1
  Sum4/1 -> Gain8/1
  Gain8/1 -> Rate Transition1/1
  Delay/1 -> Sum4/2
  x/1 -> Rate Transition/1
  Rate Transition1/1 -> dx/dt/1

== system WMMSupportingForcesGP2020a/calc_wheel_velocities_and_sideslip_angles_from_meas/Hydraulic manipulator, calculation/AnalyticTotalForces/Structure 2 (Prismatic segment)/Subsystem4 ==
  x : Inport
  Delay : Delay  DelayLength=1  InitialConditionSource=Input port
      settings: InputPortMap=u0,p4
  Gain8 : Gain  Gain=1/dT
  Rate Transition : RateTransition  OutPortSampleTime=dT
  Rate Transition1 : RateTransition
  Sum4 : Sum  Inputs=|+-
  dx/dt : Outport
  wires:
  Rate Transition/1 -> Delay/2, Delay/1, Sum4/1
  Sum4/1 -> Gain8/1
  Gain8/1 -> Rate Transition1/1
  Delay/1 -> Sum4/2
  x/1 -> Rate Transition/1
  Rate Transition1/1 -> dx/dt/1

== system WMMSupportingForcesGP2020a/calc_wheel_velocities_and_sideslip_angles_from_meas/Hydraulic manipulator, calculation/AnalyticTotalForces/Structure 2 (Prismatic segment)/Subsystem5 ==
  x : Inport
  Delay : Delay  DelayLength=1  InitialConditionSource=Input port
      settings: InputPortMap=u0,p4
  Gain8 : Gain  Gain=1/dT
  Rate Transition : RateTransition  OutPortSampleTime=dT
  Rate Transition1 : RateTransition
  Sum4 : Sum  Inputs=|+-
  dx/dt : Outport
  wires:
  Rate Transition/1 -> Delay/2, Delay/1, Sum4/1
  Sum4/1 -> Gain8/1
  Gain8/1 -> Rate Transition1/1
  Delay/1 -> Sum4/2
  x/1 -> Rate Transition/1
  Rate Transition1/1 -> dx/dt/1

== system WMMSupportingForcesGP2020a/calc_wheel_velocities_and_sideslip_angles_from_meas/Hydraulic manipulator, calculation/AnalyticTotalForces/Structure 2 (Prismatic segment)/Subsystem6 ==
  x : Inport
  Delay : Delay  DelayLength=1  InitialConditionSource=Input port
      settings: InputPortMap=u0,p4
  Gain8 : Gain  Gain=1/dT
  Rate Transition : RateTransition  OutPortSampleTime=dT
  Rate Transition1 : RateTransition
  Sum4 : Sum  Inputs=|+-
  dx/dt : Outport
  wires:
  Rate Transition/1 -> Delay/2, Delay/1, Sum4/1
  Sum4/1 -> Gain8/1
  Gain8/1 -> Rate Transition1/1
  Delay/1 -> Sum4/2
  x/1 -> Rate Transition/1
  Rate Transition1/1 -> dx/dt/1

== system WMMSupportingForcesGP2020a/calc_wheel_velocities_and_sideslip_angles_from_meas/Hydraulic manipulator, calculation/AnalyticTotalForces/Structure 2 (Revolute segment)/Subsystem1 ==
  x : Inport
  Delay : Delay  DelayLength=1  InitialConditionSource=Input port
      settings: InputPortMap=u0,p4
  Gain8 : Gain  Gain=1/dT
  Rate Transition : RateTransition  OutPortSampleTime=dT
  Rate Transition1 : RateTransition
  Sum4 : Sum  Inputs=|+-
  dx/dt : Outport
  wires:
  Rate Transition/1 -> Delay/2, Delay/1, Sum4/1
  Sum4/1 -> Gain8/1
  Gain8/1 -> Rate Transition1/1
  Delay/1 -> Sum4/2
  x/1 -> Rate Transition/1
  Rate Transition1/1 -> dx/dt/1

== system WMMSupportingForcesGP2020a/calc_wheel_velocities_and_sideslip_angles_from_meas/Hydraulic manipulator, calculation/AnalyticTotalForces/Structure 2 (Revolute segment)/Subsystem2 ==
  x : Inport
  Delay : Delay  DelayLength=1  InitialConditionSource=Input port
      settings: InputPortMap=u0,p4
  Gain8 : Gain  Gain=1/dT
  Rate Transition : RateTransition  OutPortSampleTime=dT
  Rate Transition1 : RateTransition
  Sum4 : Sum  Inputs=|+-
  dx/dt : Outport
  wires:
  Rate Transition/1 -> Delay/2, Delay/1, Sum4/1
  Sum4/1 -> Gain8/1
  Gain8/1 -> Rate Transition1/1
  Delay/1 -> Sum4/2
  x/1 -> Rate Transition/1
  Rate Transition1/1 -> dx/dt/1

== system WMMSupportingForcesGP2020a/calc_wheel_velocities_and_sideslip_angles_from_meas/Hydraulic manipulator, calculation/AnalyticTotalForces/Structure 2 (Revolute segment)/Subsystem3 ==
  x : Inport
  Delay : Delay  DelayLength=1  InitialConditionSource=Input port
      settings: InputPortMap=u0,p4
  Gain8 : Gain  Gain=1/dT
  Rate Transition : RateTransition  OutPortSampleTime=dT
  Rate Transition1 : RateTransition
  Sum4 : Sum  Inputs=|+-
  dx/dt : Outport
  wires:
  Rate Transition/1 -> Delay/2, Delay/1, Sum4/1
  Sum4/1 -> Gain8/1
  Gain8/1 -> Rate Transition1/1
  Delay/1 -> Sum4/2
  x/1 -> Rate Transition/1
  Rate Transition1/1 -> dx/dt/1

== system WMMSupportingForcesGP2020a/calc_wheel_velocities_and_sideslip_angles_from_meas/Hydraulic manipulator, calculation/AnalyticTotalForces/Structure 2 (Revolute segment)/Subsystem4 ==
  x : Inport
  Delay : Delay  DelayLength=1  InitialConditionSource=Input port
      settings: InputPortMap=u0,p4
  Gain8 : Gain  Gain=1/dT
  Rate Transition : RateTransition  OutPortSampleTime=dT
  Rate Transition1 : RateTransition
  Sum4 : Sum  Inputs=|+-
  dx/dt : Outport
  wires:
  Rate Transition/1 -> Delay/2, Delay/1, Sum4/1
  Sum4/1 -> Gain8/1
  Gain8/1 -> Rate Transition1/1
  Delay/1 -> Sum4/2
  x/1 -> Rate Transition/1
  Rate Transition1/1 -> dx/dt/1

== system WMMSupportingForcesGP2020a/calc_wheel_velocities_and_sideslip_angles_from_meas/Hydraulic manipulator, calculation/AnalyticTotalForces/Structure 2 (Revolute segment)/Subsystem5 ==
  x : Inport
  Delay : Delay  DelayLength=1  InitialConditionSource=Input port
      settings: InputPortMap=u0,p4
  Gain8 : Gain  Gain=1/dT
  Rate Transition : RateTransition  OutPortSampleTime=dT
  Rate Transition1 : RateTransition
  Sum4 : Sum  Inputs=|+-
  dx/dt : Outport
  wires:
  Rate Transition/1 -> Delay/2, Delay/1, Sum4/1
  Sum4/1 -> Gain8/1
  Gain8/1 -> Rate Transition1/1
  Delay/1 -> Sum4/2
  x/1 -> Rate Transition/1
  Rate Transition1/1 -> dx/dt/1

== system WMMSupportingForcesGP2020a/calc_wheel_velocities_and_sideslip_angles_from_meas/Hydraulic manipulator, calculation/AnalyticTotalForces/Structure 2 (Revolute segment)/Subsystem6 ==
  x : Inport
  Delay : Delay  DelayLength=1  InitialConditionSource=Input port
      settings: InputPortMap=u0,p4
  Gain8 : Gain  Gain=1/dT
  Rate Transition : RateTransition  OutPortSampleTime=dT
  Rate Transition1 : RateTransition
  Sum4 : Sum  Inputs=|+-
  dx/dt : Outport
  wires:
  Rate Transition/1 -> Delay/2, Delay/1, Sum4/1
  Sum4/1 -> Gain8/1
  Gain8/1 -> Rate Transition1/1
  Delay/1 -> Sum4/2
  x/1 -> Rate Transition/1
  Rate Transition1/1 -> dx/dt/1

== system WMMSupportingForcesGP2020a/calc_wheel_velocities_and_sideslip_angles_from_meas/Hydraulic manipulator, calculation/AnalyticTotalForces/Structure 2 (Revolute segment)/Subsystem7 ==
  x : Inport
  Delay : Delay  DelayLength=1  InitialConditionSource=Input port
      settings: InputPortMap=u0,p4
  Gain8 : Gain  Gain=1/dT
  Rate Transition : RateTransition  OutPortSampleTime=dT
  Rate Transition1 : RateTransition
  Sum4 : Sum  Inputs=|+-
  dx/dt : Outport
  wires:
  Rate Transition/1 -> Delay/2, Delay/1, Sum4/1
  Sum4/1 -> Gain8/1
  Gain8/1 -> Rate Transition1/1
  Delay/1 -> Sum4/2
  x/1 -> Rate Transition/1
  Rate Transition1/1 -> dx/dt/1

== system WMMSupportingForcesGP2020a/calc_wheel_velocities_and_sideslip_angles_from_meas/Hydraulic manipulator, calculation/AnalyticTotalForces/Structure 2 (Revolute segment)/Subsystem8 ==
  x : Inport
  Delay : Delay  DelayLength=1  InitialConditionSource=Input port
      settings: InputPortMap=u0,p4
  Gain8 : Gain  Gain=1/dT
  Rate Transition : RateTransition  OutPortSampleTime=dT
  Rate Transition1 : RateTransition
  Sum4 : Sum  Inputs=|+-
  dx/dt : Outport
  wires:
  Rate Transition/1 -> Delay/2, Delay/1, Sum4/1
  Sum4/1 -> Gain8/1
  Gain8/1 -> Rate Transition1/1
  Delay/1 -> Sum4/2
  x/1 -> Rate Transition/1
  Rate Transition1/1 -> dx/dt/1

== system WMMSupportingForcesGP2020a/calc_wheel_velocities_and_sideslip_angles_from_meas/Hydraulic manipulator, calculation/AnalyticVelocities/Structure 1/GeomPropS1 ==
  note: Get inputs...
  note: Pass to outputs...
  note: Process data...
  note: Create new buses...
  q1 : Inport
  Bus Creator : BusCreator  Inputs=q1,x1,q11,q12,dq1,dx1,dq11,dq12
  LiftPistonStroke : Subsystem
  Subsystem : Subsystem
  Subsystem1 : Subsystem
  Subsystem2 : Subsystem
  q11-angle : Subsystem
  q12-angle : Subsystem
  q1Derivative : Subsystem
  GeomProp_S1 : Outport
  wires:
  q1/1 -> [q1]  "q1"
  [q1] -> LiftPistonStroke/1(q1[rad])  "q1"
  LiftPistonStroke/1(x1[m]) -> [x1]  "x1"
  [x1] -> q11-angle/1(x1)  "x1"
  [x1] -> q12-angle/1(x1)  "x1"
  [dq1] -> Bus Creator/5  "dq1"
  q12-angle/1(q12) -> [q12]  "q12"
  [q12] -> Bus Creator/4  "q12"
  [q1] -> Bus Creator/1  "q1"
  [x1] -> Bus Creator/2  "x1"
  q11-angle/1(q11) -> [q11]  "q11"
  [q11] -> Bus Creator/3  "q11"
  [dx1] -> Bus Creator/6  "dx1"
  [dq12] -> Bus Creator/8  "dq12"
  [dq11] -> Bus Creator/7  "dq11"
  Bus Creator/1 -> [GeomPropS1]
  [GeomPropS1] -> GeomProp_S1/1
  [q1] -> q1Derivative/1(q1)  "q1"
  q1Derivative/1(dq1) -> [dq1]  "dq1"
  [dq1] -> Subsystem/1(dq1)  "dq1"
  [x1] -> Subsystem/2(x1)  "x1"
  [q1] -> Subsystem/3(q1)  "q1"
  Subsystem/1(dx1) -> [dx1]  "dx1"
  [dx1] -> Subsystem1/3(dx1)  "dx1"
  [x1] -> Subsystem1/1(x1)  "x1"
  [q11] -> Subsystem1/2(q11)  "q11"
  Subsystem1/1(dq11) -> [dq11]  "dq11"
  Subsystem2/1(dq12) -> [dq12]  "dq12"
  [dx1] -> Subsystem2/3(dx1)  "dx1"
  [x1] -> Subsystem2/1(x1)  "x1"
  [q12] -> Subsystem2/2(q12)  "q12"

== system WMMSupportingForcesGP2020a/calc_wheel_velocities_and_sideslip_angles_from_meas/Hydraulic manipulator, calculation/AnalyticVelocities/Structure 1/PosVecsS1 ==
  note: Select from existing buses...
  note: Pass to outputs...
  note: Create new buses...
  note: Process data...
  note: Form time-varying position vectors...
  note: Get inputs...
  GeomProp_CC1 : Inport
  B11_r_B11Tc1 : Constant  Value=B11_r_B11Tc1
  B31_r_B31B41 : MATLAB Function  TreatAsAtomicUnit=on
  B41_r_B41Tc1 : Constant  Value=B41_r_B41Tc1
  Bc1_r_Bc1B1 : Constant  Value=W_r_WBc1
  Bc1_r_Bc1B11 : Constant  Value=Bc1_r_Bc1B11
  Bc1_r_Bc1B31 : Constant  Value=Bc1_r_Bc1B31
  Bus Creator : BusCreator  Inputs=Tc1_r_Tc1Bc2,B41_r_B41Tc1,B31_r_B31B41,Bc1_r_Bc1B31,B11_r_B11Tc1,Bc1_r_Bc1B11,W_r_WBc1
  Bus Selector : BusSelector  OutputSignals=x1
  Tc1_r_Tc1Bc2 : Constant  Value=Tc1_r_Tc1Bc2
  PosVecs_S1 : Outport
  wires:
  Bus Creator/1 -> [PosVecsS1]
  GeomProp_CC1/1 -> [GeomPropCC1]  "GeomProp_CC1"
  [GeomPropCC1] -> Bus Selector/1
  Tc1_r_Tc1Bc2/1 -> [rTc1Bc2]  "Tc1_r_Tc1Bc2"
  [rTc1Bc2] -> Bus Creator/1  "Tc1_r_Tc1Bc2"
  B41_r_B41Tc1/1 -> [rB41Tc1]  "B41_r_B41Tc1"
  [rB41Tc1] -> Bus Creator/2  "B41_r_B41Tc1"
  B31_r_B31B41/1(B31_r_B31B41) -> [rB31B41]  "B31_r_B31B41"
  [rB31B41] -> Bus Creator/3  "B31_r_B31B41"
  Bc1_r_Bc1B31/1 -> [rBc1B31]  "Bc1_r_Bc1B31"
  B11_r_B11Tc1/1 -> [rB11Tc1]  "B11_r_B11Tc1"
  Bc1_r_Bc1B11/1 -> [rBc1B11]  "Bc1_r_Bc1B11"
  [rBc1B31] -> Bus Creator/4  "Bc1_r_Bc1B31"
  [rB11Tc1] -> Bus Creator/5  "B11_r_B11Tc1"
  [rBc1B11] -> Bus Creator/6  "Bc1_r_Bc1B11"
  Bus Selector/1 -> [x1]  "<x1>"
  [x1] -> B31_r_B31B41/1(x1)
  [PosVecsS1] -> PosVecs_S1/1  "PosVecs_S1"
  [rWBc1] -> Bus Creator/7  "W_r_WBc1"
  Bc1_r_Bc1B1/1 -> [rWBc1]  "W_r_WBc1"

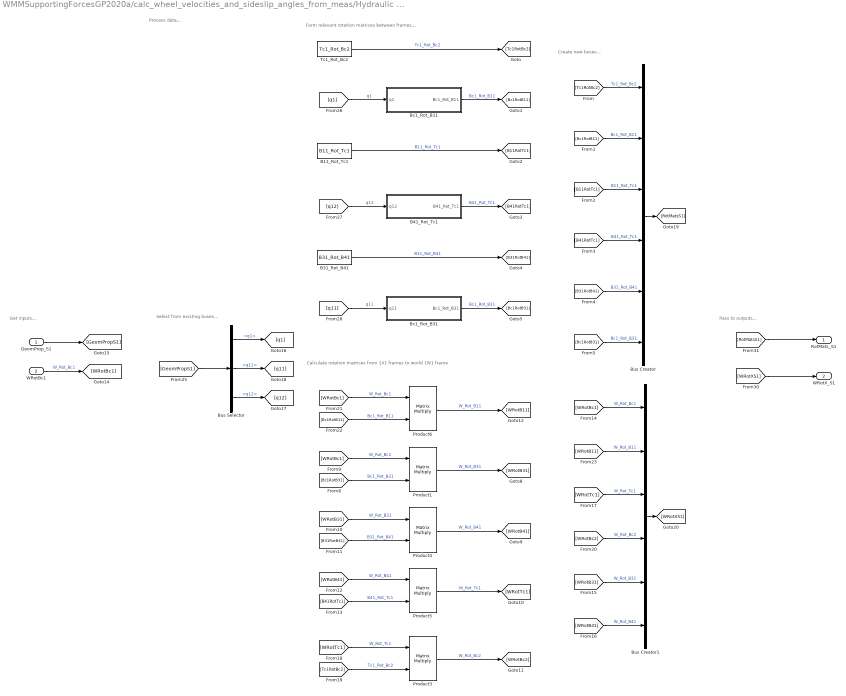
== system WMMSupportingForcesGP2020a/calc_wheel_velocities_and_sideslip_angles_from_meas/Hydraulic manipulator, calculation/AnalyticVelocities/Structure 1/RotMatsS1 ==
  note: Create new buses...
  note: Pass to outputs...
  note: Get inputs...
  note: Process data...
  note: Select from existing buses...
  note: Form relevant rotation matrices between frames...
  note: Calculate rotation matrices from {X} frames to world {W} frame
  GeomProp_S1 : Inport
  WRotBc1 : Inport  Port=2
  B11_Rot_Tc1 : Constant  Value=B11_Rot_Tc1
  B31_Rot_B41 : Constant  Value=B31_Rot_B41
  B41_Rot_Tc1 : MATLAB Function  TreatAsAtomicUnit=on
  Bc1_Rot_B11 : MATLAB Function  TreatAsAtomicUnit=on
  Bc1_Rot_B31 : MATLAB Function  TreatAsAtomicUnit=on
  Bus Creator : BusCreator  Inputs=6
  Bus Creator1 : BusCreator  Inputs=W_Rot_Bc1,W_Rot_B11,W_Rot_Tc1,W_Rot_Bc2,W_Rot_B31,W_Rot_B41
  Bus Selector : BusSelector  OutputSignals=q1,q11,q12
  Product{1,3..6} (5 alike) : Product  Multiplication=Matrix(*)
  Tc1_Rot_Bc2 : Constant  Value=Tc1_Rot_Bc2
  RotMats_S1 : Outport
  WRotX_S1 : Outport  Port=2
  wires:
  [Tc1RotBc2] -> Bus Creator/1  "Tc1_Rot_Bc2"
  Tc1_Rot_Bc2/1 -> [Tc1RotBc2]  "Tc1_Rot_Bc2"
  [Bc1RotB11] -> Bus Creator/2  "Bc1_Rot_B11"
  Bc1_Rot_B11/1(Bc1_Rot_B11) -> [Bc1RotB11]  "Bc1_Rot_B11"
  [B11RotTc1] -> Bus Creator/3  "B11_Rot_Tc1"
  B11_Rot_Tc1/1 -> [B11RotTc1]  "B11_Rot_Tc1"
  B41_Rot_Tc1/1(B41_Rot_Tc1) -> [B41RotTc1]  "B41_Rot_Tc1"
  [B41RotTc1] -> Bus Creator/4  "B41_Rot_Tc1"
  B31_Rot_B41/1 -> [B31RotB41]  "B31_Rot_B41"
  [B31RotB41] -> Bus Creator/5  "B31_Rot_B41"
  Bc1_Rot_B31/1(Bc1_Rot_B31) -> [Bc1RotB31]  "Bc1_Rot_B31"
  [Bc1RotB31] -> Bus Creator/6  "Bc1_Rot_B31"
  [WRotBc1] -> Product1/1  "W_Rot_Bc1"
  [Bc1RotB31] -> Product1/2  "Bc1_Rot_B31"
  Product1/1 -> [WRotB31]  "W_Rot_B31"
  [WRotB31] -> Product4/1  "W_Rot_B31"
  [B31RotB41] -> Product4/2  "B31_Rot_B41"
  Product4/1 -> [WRotB41]  "W_Rot_B41"
  Product5/1 -> [WRotTc1]  "W_Rot_Tc1"
  [B41RotTc1] -> Product5/2  "B41_Rot_Tc1"
  [WRotB41] -> Product5/1  "W_Rot_B41"
  [WRotTc1] -> Product3/1  "W_Rot_Tc1"
  [Tc1RotBc2] -> Product3/2  "Tc1_Rot_Bc2"
  Product3/1 -> [WRotBc2]  "W_Rot_Bc2"
  [WRotBc1] -> Product6/1  "W_Rot_Bc1"
  [Bc1RotB11] -> Product6/2  "Bc1_Rot_B11"
  Product6/1 -> [WRotB11]  "W_Rot_B11"
  [WRotB11] -> Bus Creator1/2  "W_Rot_B11"
  [WRotBc1] -> Bus Creator1/1  "W_Rot_Bc1"
  [WRotB41] -> Bus Creator1/6  "W_Rot_B41"
  [WRotB31] -> Bus Creator1/5  "W_Rot_B31"
  [WRotBc2] -> Bus Creator1/4  "W_Rot_Bc2"
  [WRotTc1] -> Bus Creator1/3  "W_Rot_Tc1"
  WRotBc1/1 -> [WRotBc1]  "W_Rot_Bc1"
  GeomProp_S1/1 -> [GeomPropS1]
  [GeomPropS1] -> Bus Selector/1
  Bus Selector/1 -> [q1]  "<q1>"
  Bus Selector/3 -> [q12]  "<q12>"
  Bus Selector/2 -> [q11]  "<q11>"
  [q1] -> Bc1_Rot_B11/1(q1)  "q1"
  [q12] -> B41_Rot_Tc1/1(q12)  "q12"
  [q11] -> Bc1_Rot_B31/1(q11)  "q11"
  Bus Creator/1 -> [RotMatsS1]
  Bus Creator1/1 -> [WRotXS1]
  [WRotXS1] -> WRotX_S1/1
  [RotMatsS1] -> RotMats_S1/1

== system WMMSupportingForcesGP2020a/calc_wheel_velocities_and_sideslip_angles_from_meas/Hydraulic manipulator, calculation/AnalyticVelocities/Structure 1/UMatsS1 ==
  note: Get inputs...
  note: Pass to outputs...
  note: Form new buses...
  note: Process data...
  note: Form relevant velocity/force transformation matrices...
  note: Select form existing buses...
  PosVecs_S1 : Inport
  RotMats_S1 : Inport  Port=2
  B11_U_Tc1 : MATLAB Function  TreatAsAtomicUnit=on
  B31_U_B41 : MATLAB Function  TreatAsAtomicUnit=on
  B41_U_Tc1 : MATLAB Function  TreatAsAtomicUnit=on
  Bc1_U_B11 : MATLAB Function  TreatAsAtomicUnit=on
  Bc1_U_B31 : MATLAB Function  TreatAsAtomicUnit=on
  Bus Creator : BusCreator  Inputs=6
  Bus Selector : BusSelector  OutputSignals=Tc1_r_Tc1Bc2,B41_r_B41Tc1,B31_r_B31B41,Bc1_r_Bc1B31,B11_r_B11Tc1,Bc1_r_Bc1B11
  Bus Selector1 : BusSelector  OutputSignals=Tc1_Rot_Bc2,B41_Rot_Tc1,B31_Rot_B41,Bc1_Rot_B31,B11_Rot_Tc1,Bc1_Rot_B11
  Tc1_U_Bc2 : MATLAB Function  TreatAsAtomicUnit=on
  UMat_S1 : Outport
  wires:
  Bus Selector/2 -> [rB41Tc1]  "<B41_r_B41Tc1>"
  [rB41Tc1] -> B41_U_Tc1/1(B41_r_B41Tc1)
  Bus Selector/3 -> [rB31B41]  "<B31_r_B31B41>"
  Bus Selector/5 -> [rB11Tc1]  "<B11_r_B11Tc1>"
  Bus Selector/4 -> [rBc1B31]  "<Bc1_r_Bc1B31>"
  Bus Selector/6 -> [rBc1B11]  "<Bc1_r_Bc1B11>"
  [rBc1B11] -> Bc1_U_B11/1(Bc1_r_Bc1B11)
  [rB11Tc1] -> B11_U_Tc1/1(B11_r_B11Tc1)
  [rBc1B31] -> Bc1_U_B31/1(Bc1_r_Bc1B31)
  [rB31B41] -> B31_U_B41/1(B31_r_B31B41)
  Bus Selector1/2 -> [B41RotTc1]  "<B41_Rot_Tc1>"
  Bus Selector1/3 -> [B31RotB41]  "<B31_Rot_B41>"
  Bus Selector1/4 -> [Bc1RotB31]  "<Bc1_Rot_B31>"
  Bus Selector1/5 -> [B11RotTc1]  "<B11_Rot_Tc1>"
  Bus Selector1/6 -> [Bc1RotB11]  "<Bc1_Rot_B11>"
  [Bc1RotB11] -> Bc1_U_B11/2(Bc1_Rot_B11)
  [B11RotTc1] -> B11_U_Tc1/2(B11_Rot_Tc1)
  [Bc1RotB31] -> Bc1_U_B31/2(Bc1_Rot_B31)
  [B31RotB41] -> B31_U_B41/2(B31_Rot_B41)
  [B41RotTc1] -> B41_U_Tc1/2(B41_Rot_Tc1)
  Bus Selector1/1 -> [Tc1RotBc2]  "<Tc1_Rot_Bc2>"
  Bus Selector/1 -> [rTc1Bc2]  "<Tc1_r_Tc1Bc2>"
  [Tc1RotBc2] -> Tc1_U_Bc2/2(Tc1_Rot_Bc2)
  [rTc1Bc2] -> Tc1_U_Bc2/1(Tc1_r_Tc1Bc2)
  Bus Creator/1 -> [UMatS1]  "UMat_S1"
  PosVecs_S1/1 -> [PosVecsS1]
  [PosVecsS1] -> Bus Selector/1
  RotMats_S1/1 -> [RotMatsS1]
  [RotMatsS1] -> Bus Selector1/1
  Tc1_U_Bc2/1(Tc1_U_Bc2) -> [Tc1UBc2]  "Tc1_U_Bc2"
  [Tc1UBc2] -> Bus Creator/1  "Tc1_U_Bc2"
  B41_U_Tc1/1(B41_U_Tc1) -> [B41UTc1]  "B41_U_Tc1"
  [B41UTc1] -> Bus Creator/2  "B41_U_Tc1"
  B31_U_B41/1(B31_U_B41) -> [B31UB41]  "B31_U_B41"
  [B31UB41] -> Bus Creator/3  "B31_U_B41"
  Bc1_U_B31/1(Bc1_U_B31) -> [Bc1UB31]  "Bc1_U_B31"
  B11_U_Tc1/1(B11_U_Tc1) -> [B11UTc1]  "B11_U_Tc1"
  Bc1_U_B11/1(Bc1_U_B11) -> [Bc1UB11]  "Bc1_U_B11"
  [Bc1UB31] -> Bus Creator/4  "Bc1_U_B31"
  [B11UTc1] -> Bus Creator/5  "B11_U_Tc1"
  [Bc1UB11] -> Bus Creator/6  "Bc1_U_B11"
  [UMatS1] -> UMat_S1/1
